simulink model "two_link_model_env"  (R2021a)
settings: Solver=VariableStepAuto  StartTime=0.0  StopTime=10.0  RelTol=1e-3
undefined symbols (not defined in the file): a_1, a_2, F, K, o_r
settings Model: Creator=frida  LastModifiedBy=frida

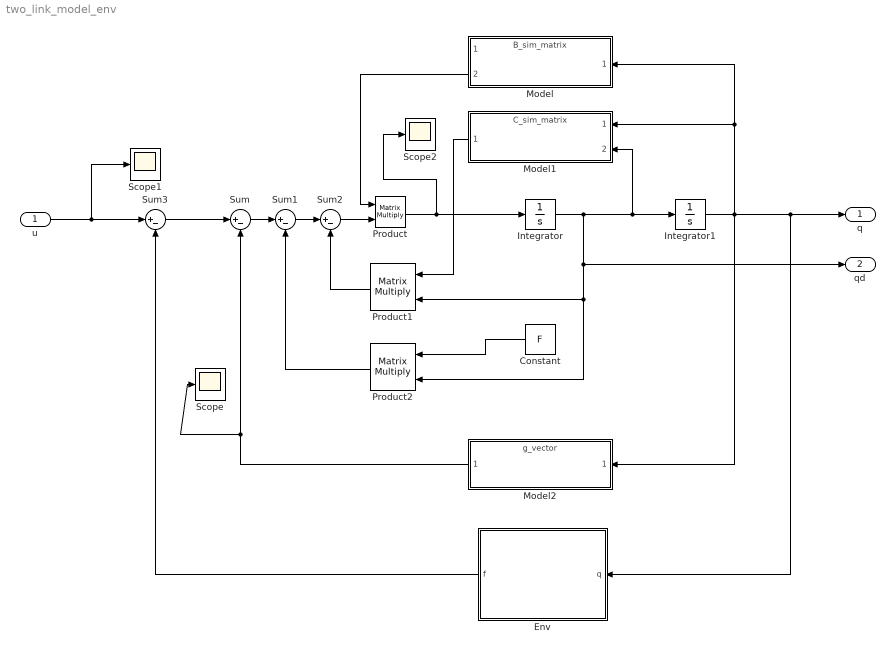
== system two_link_model_env ==
  u : Inport  PortDimensions=2
  Constant : Constant  Value=F
  Env : Subsystem
  Integrator : Integrator
  Integrator1 : Integrator
  Model : ModelReference  ModelNameDialog=B_sim_matrix.slx  SimulationMode=Normal  ModelReferenceVersion=1.6
  Model1 : ModelReference  ModelNameDialog=C_sim_matrix.slx  SimulationMode=Normal  ModelReferenceVersion=1.2
  Model2 : ModelReference  ModelNameDialog=g_vector.slx  SimulationMode=Normal  ModelReferenceVersion=1.8
  Product : Product  Multiplication=Matrix(*)
  Product1 : Product  Multiplication=Matrix(*)
  Product2 : Product  Multiplication=Matrix(*)
  Scope : Scope
  Scope1 : Scope
  Scope2 : Scope
  Sum{,1..3} (4 alike) : Sum  Inputs=|+-
  q : Outport  PortDimensions=2
  qd : Outport  Port=2  PortDimensions=2
  wires:
  Sum3/1 -> Sum/1
  Product1/1 -> Sum2/2
  Sum2/1 -> Product/2
  Product/1 -> Scope2/1, Integrator/1
  Model2/1 -> Scope/1, Sum/2
  Integrator1/1 -> Model2/1, Env/1(q), q/1, Model/1, Model1/1
  Model1/1 -> Product1/1
  Sum/1 -> Sum1/1
  Constant/1 -> Product2/1
  Sum1/1 -> Sum2/1
  Product2/1 -> Sum1/2
  Integrator/1 -> qd/1, Product2/2, Product1/2, Model1/2, Integrator1/1
  Model/2 -> Product/1
  Env/1(f) -> Sum3/2
  u/1 -> Scope1/1, Sum3/1

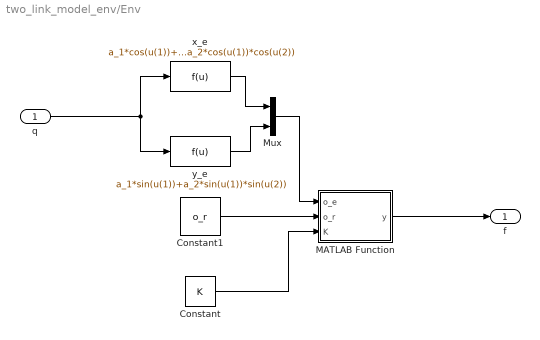
== system two_link_model_env/Env ==
  q : Inport
  Constant : Constant  Value=K
  Constant1 : Constant  Value=o_r
  MATLAB Function : MATLAB Function  TreatAsAtomicUnit=on
  Mux : Mux  Inputs=2
  x_e : Fcn  Expr=a_1*cos(u(1))+a_2*cos(u(1))*cos(u(2))
  y_e : Fcn  Expr=a_1*sin(u(1))+a_2*sin(u(1))*sin(u(2))
  f : Outport
  wires:
  Constant1/1 -> MATLAB Function/2(o_r)
  Constant/1 -> MATLAB Function/3(K)
  MATLAB Function/1(y) -> f/1
  q/1 -> y_e/1, x_e/1
  y_e/1 -> Mux/2
  x_e/1 -> Mux/1
  Mux/1 -> MATLAB Function/1(o_e)

== matlab function two_link_model_env/Env/MATLAB Function ==
  data: o_e input; y output; o_r input; K input
function y = fcn(o_e, o_r, K)
if o_e(1) < o_r(1)
    y = [0; 0];
else
    % In this case the K matrix is a 
    % (2 x 2) matrix where only k_x is defined, 
    % therefore the returned y contains 
    % only forces in x-direction
    y = K*[o_e(1)-o_r(1); o_e(2)-o_r(2)];
end
